simulink model "piezo_GO_RCvar_p48_3"  (R2022a)
settings: Solver=VariableStepAuto  StartTime=0.0  StopTime=150  RelTol=1e-3
undefined symbols (not defined in the file or in its folder): Kc, Kr, Rc, Rct
libraries: fl_lib x7, nesl_utility x6, spsTriangleGeneratorLib x1, ee_lib x1
settings Model: Creator=sasikada  LastModifiedBy=sasikada

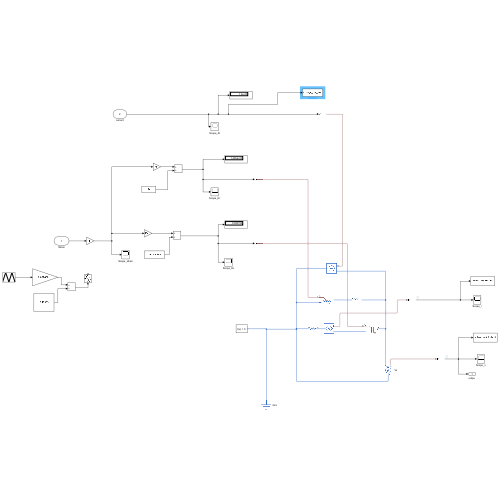
[thumbnail: Simulink's stored preview of the top-level diagram]
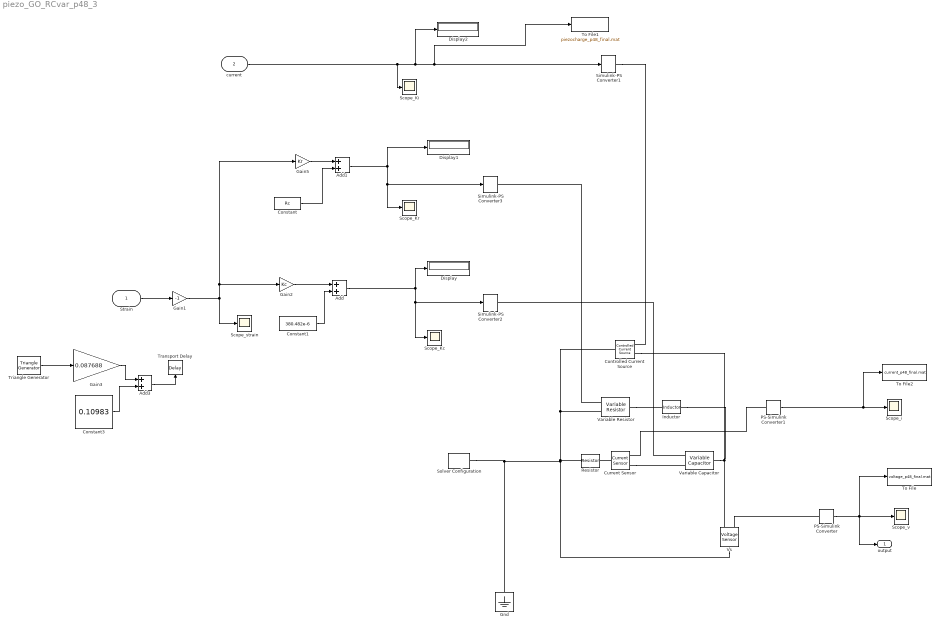
== system piezo_GO_RCvar_p48_3 ==
  Strain : Inport
  current : Inport  Port=2
  Add : Sum
  Add1 : Sum
  Add3 : Sum
  Constant : Constant  Value=Rc
  Constant1 : Constant  Value=380.482e-6
  Constant3 : Constant  Value=0.10983
  Controlled Current Source : fl_lib/Electrical/Electrical Sources/Controlled Current Source
      settings: SourceProductBaseCode=PW,SS,VE
  Current Sensor : fl_lib/Electrical/Electrical Sensors/Current Sensor
      settings: SourceProductBaseCode=PW,SS,VE
  Display : Display
  Display1 : Display
  Display2 : Display
  Gain1 : Gain  Gain=-1
  Gain2 : Gain  Gain=Kc
  Gain3 : Gain  Gain=0.087688
  Gain5 : Gain  Gain=Kr
  Gnd : fl_lib/Electrical/Electrical Elements/Electrical Reference
      settings: SourceProductBaseCode=PW,SS,VE
  Inductor : fl_lib/Electrical/Electrical Elements/Inductor  l=L H  r=0 Ohm  g=1e-9 1/Ohm  i_specify=off  i_priority=None  i=0 A  i_nominal_specify=off  i_nominal_unit=A  i_nominal_value=1  v_specify=off  v_priority=None  v=0 V  v_nominal_specify=off  v_nominal_unit=V  v_nominal_value=1  i_L_specify=off  i_L_priority=High  i_L=0 A  i_L_nominal_specify=off  i_L_nominal_unit=A  i_L_nominal_value=1
      settings: SourceProductBaseCode=PW,SS,VE
  PS-Simulink Converter : nesl_utility/PS-Simulink Converter  PhysicalDomain=network_engine_domain  SubClassName=ps_output  LeftPortType=input  RightPortType=output  PseudoPeriodic=off  Frequencies=[]  VectorFormat=1-D array  Unit=V  AffineConversion=off
      settings: SourceProductBaseCode=SS,PW,VE
  PS-Simulink Converter1 : nesl_utility/PS-Simulink Converter  PhysicalDomain=network_engine_domain  SubClassName=ps_output  LeftPortType=input  RightPortType=output  PseudoPeriodic=off  Frequencies=[]  VectorFormat=1-D array  Unit=A  AffineConversion=off
      settings: SourceProductBaseCode=SS,PW,VE
  Resistor : fl_lib/Electrical/Electrical Elements/Resistor  R=Rct Ohm  i_specify=off  i_priority=None  i=0 A  i_nominal_specify=off  i_nominal_unit=A  i_nominal_value=1  v_specify=off  v_priority=None  v=0 V  v_nominal_specify=off  v_nominal_unit=V  v_nominal_value=1
      settings: SourceProductBaseCode=PW,SS,VE
  Scope_Kc : Scope
  Scope_Ki : Scope
  Scope_Kr : Scope
  Scope_i : Scope
  Scope_strain : Scope
  Scope_v : Scope
  Simulink-PS Converter1 : nesl_utility/Simulink-PS Converter  PhysicalDomain=network_engine_domain  SubClassName=ps_input  LeftPortType=input  RightPortType=output  PseudoPeriodic=off  Frequencies=[]  NoiseDistribution=none  NoiseParameters=[]  Unit=A  AffineConversion=on  FilteringAndDerivatives=zero  SimscapeFilterOrder=1  InputFilterTimeConstant=0.001  UdotUserProvided=1
      settings: SourceProductBaseCode=SS,PW,VE
  Simulink-PS Converter2 : nesl_utility/Simulink-PS Converter  PhysicalDomain=network_engine_domain  SubClassName=ps_input  LeftPortType=input  RightPortType=output  PseudoPeriodic=off  Frequencies=[]  NoiseDistribution=none  NoiseParameters=[]  Unit=F  AffineConversion=on  FilteringAndDerivatives=zero  SimscapeFilterOrder=1  InputFilterTimeConstant=0.001  UdotUserProvided=1
      settings: SourceProductBaseCode=SS,PW,VE
  Simulink-PS Converter3 : nesl_utility/Simulink-PS Converter  PhysicalDomain=network_engine_domain  SubClassName=ps_input  LeftPortType=input  RightPortType=output  PseudoPeriodic=off  Frequencies=[]  NoiseDistribution=none  NoiseParameters=[]  Unit=Ohm  AffineConversion=on  FilteringAndDerivatives=zero  SimscapeFilterOrder=1  InputFilterTimeConstant=0.001  UdotUserProvided=1
      settings: SourceProductBaseCode=SS,PW,VE
  Solver Configuration : nesl_utility/Solver Configuration  PhysicalDomain=network_engine_domain  SubClassName=solver  LeftPortType=input  RightPortType=generic  Tones=[]  Harmonics=[]  SimulateNoise=off  Profile=off  UseLocalSampling=off  EnableSwitchedLinearOptims=on  FrequencyDomain=off  UseCCode=off  RelTol=0.001  AbsTol=1e-06  MinStep=1e-09  ToWorkspace=off  RevertToSquareIcSolve=off  NumHomotopyIterations=100  PhasorMode=off  PhasorModeNumHarmonics=1  IndexReductionMethod=DerivativeReplacement  DoDC=off  ResidualTolerance=1e-09  UseLocalSolver=on  LocalSolverChoice=NE_BACKWARD_EULER_ADVANCER  LocalSolverSampleTime=0.04  DoFixedCost=on  MaxNonlinIter=3  MaxModeIter=2  ComputeImpulses=off  ImpulseIterations=2  LinearAlgebra=Sparse  LinearAlgebraNumThread=0  EquationFormulation=NE_TIME_EF  DelaysMemoryBudget=1024  AutomaticFiltering=off  FilteringTimeConstant=0.1  PartitionStorageMethod=AS_NEEDED  PartitionMemoryBudget=1024  PartitionMethod=FAST
      settings: SourceProductBaseCode=SS,PW,VE
  To File : ToFile  Filename=voltage_p48_final.mat  MatrixName=sol
  To File1 : ToFile  Filename=piezocharge_p48_final.mat  MatrixName=piezo
  To File2 : ToFile  Filename=current_p48_final.mat  MatrixName=current
  Transport Delay : TransportDelay  DelayTime=0  InitialOutput=-0.5*10^(-4)
  Triangle Generator : spsTriangleGeneratorLib/Triangle Generator  Freq=0.0435  Phase=0  Ts=0
  Variable Capacitor : ee_lib/Passive/Variable Capacitor  prm=2  Cmin=10e-9 F  r=1e-6 Ohm  v0=V_ini V  q0=0 c
      settings: SourceProductBaseCode=PS  InternalSimscapePortConfiguration="{\"Bottom\":[],\"Left\":[{\"id\":\"C\",\"label\":\"C\",\"type\":\"input\"},{\"id\":\"p\",\"label\":\"+\",\"type\":\"foundation.electrical.electrical\"}],\"Right\":[{\"id\":\"n\",\"label\":\"-\",\"type\":\"foundation.electrical.electrical\"}],\"Top\":[]}"
  Variable Resistor : fl_lib/Electrical/Electrical Elements/Variable Resistor  Rmin=0 Ohm  i_specify=off  i_priority=None  i=0 A  i_nominal_specify=off  i_nominal_unit=A  i_nominal_value=1  v_specify=off  v_priority=None  v=0 V  v_nominal_specify=off  v_nominal_unit=V  v_nominal_value=1
      settings: SourceProductBaseCode=PW,SS,VE
  Vs : fl_lib/Electrical/Electrical Sensors/Voltage Sensor
      settings: SourceProductBaseCode=PW,SS,VE
  output : Outport
  wires:
  current/1 -> Scope_Ki/1, Display2/1, To File1/1, Simulink-PS Converter1/1
  Triangle Generator/1 -> Gain3/1
  Constant3/1 -> Add3/2
  PS-Simulink Converter1/1 -> Scope_i/1, To File2/1
  Gain3/1 -> Add3/1
  Add3/1 -> Transport Delay/1
  PS-Simulink Converter/1 -> Scope_v/1, To File/1, output/1
  Strain/1 -> Gain1/1
  Gain5/1 -> Add1/1
  Add1/1 -> Scope_Kr/1, Simulink-PS Converter3/1, Display1/1
  Gain2/1 -> Add/1
  Constant1/1 -> Add/2
  Add/1 -> Display/1, Scope_Kc/1, Simulink-PS Converter2/1
  Gain1/1 -> Gain2/1, Gain5/1, Scope_strain/1
  Constant/1 -> Add1/2
  connections:
  Variable Capacitor/LConn1 -- Simulink-PS Converter2/RConn1
  Vs/RConn1 -- PS-Simulink Converter/LConn1
  Variable Resistor/LConn1 -- Simulink-PS Converter3/RConn1
  PS-Simulink Converter1/LConn1 -- Current Sensor/RConn1
  Variable Resistor/RConn1 -- Inductor/LConn1
  Simulink-PS Converter1/RConn1 -- Controlled Current Source/RConn1
  Vs/RConn2 -- Controlled Current Source/RConn2 -- Inductor/RConn1 -- Variable Capacitor/RConn1
  Variable Resistor/LConn2 -- Controlled Current Source/LConn1 -- Resistor/LConn1 -- Vs/LConn1 -- Gnd/LConn1 -- Solver Configuration/RConn1
  Current Sensor/LConn1 -- Resistor/RConn1
  Current Sensor/RConn2 -- Variable Capacitor/LConn2
